simulink model "simple_system"  (R2024a)
settings: Solver=VariableStepAuto  StartTime=0.0  StopTime=10.0  RelTol=1e-3
values from neighbouring files (symbols this model uses):
  c = 3.0    [simplesystemDD.sldd]
  k = 5.0    [simplesystemDD.sldd]
  m = 2.0    [simplesystemDD.sldd]
settings Model: DataDictionary=simplesystemDD.sldd  Creator=The MathWorks, Inc.  LastModifiedBy=grouleau
settings SolverCC: AlgebraicLoopSolver=TrustRegion
settings DataIOCC: ReturnWorkspaceOutputs=off
settings OptimizationCC: ReuseModelBlockBuffer=off
settings DebuggingCC: UnconnectedInputMsg=warning  UnconnectedOutputMsg=warning  UnconnectedLineMsg=warning  PregeneratedLibrarySubsystemCodeDiagnostic=none  ArithmeticOperatorsInVariantConditions=warning
settings ModelReferenceCC: EnableRefExpFcnMdlSchedulingChecks=on
settings SFSimCC: SimUseLocalCustomCode=off  CustomCodeUndefinedFunction=UseInterfaceOnly
settings RTWCC: RTWUseLocalCustomCode=off  GPUComputeCapability=3.5

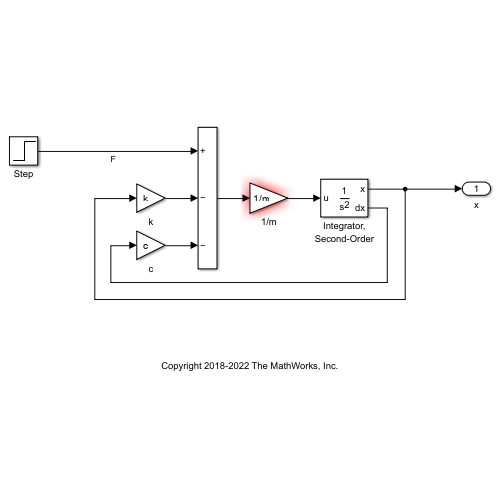
[thumbnail: Simulink's stored preview of the top-level diagram]
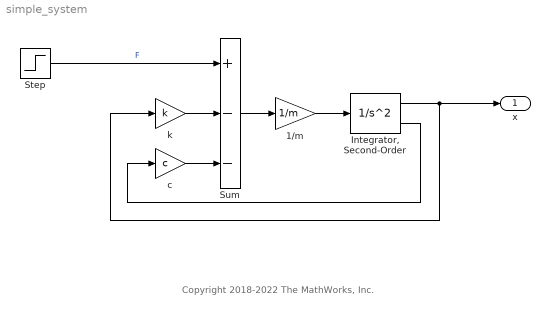
== system simple_system ==
  note: Copyright 2018-2022 The MathWorks, Inc.
  1/m : Gain  Gain=1/m
  "Integrator, Second-Order" : SecondOrderIntegrator
  Step : Step  SampleTime=0
  Sum : Sum  Inputs=+--
  c : Gain  Gain=c
  k : Gain  Gain=k
  x : Outport
  wires:
  Step/1 -> Sum/1  "F"
  c/1 -> Sum/3
  k/1 -> Sum/2
  Sum/1 -> 1/m/1
  "Integrator, Second-Order"/2 -> c/1
  "Integrator, Second-Order"/1 -> x/1, k/1
  1/m/1 -> "Integrator, Second-Order"/1
